simulink model "parte3_ex2"  (R2021b)
settings: Solver=VariableStepAuto  StartTime=0.0  StopTime=10  RelTol=1e-3
values from neighbouring files (symbols this model uses):
  h = 0.03    [parte3_script.m]
  Jm = 1.3475e-6    (= 1.3475e-06)    [parte3_script.m]
  Ke = 0.0159    [parte3_script.m]
  Kf = 0.000001176    (= 1.176e-06)    [parte3_script.m]
  L = Laa(2:end)    [parte3_script.m]
  L1 = -Laa(1)    [parte3_script.m]
  La = 0    [parte3_script.m]
  Lc = L1/(1-polo_i)    [parte3_script.m]
  Ra = 8    [parte3_script.m]
undefined symbols (not defined in the file or in its folder): DiscIntNeverNeededParam
settings Model: Creator=Dylan  LastModifiedBy=Dylan

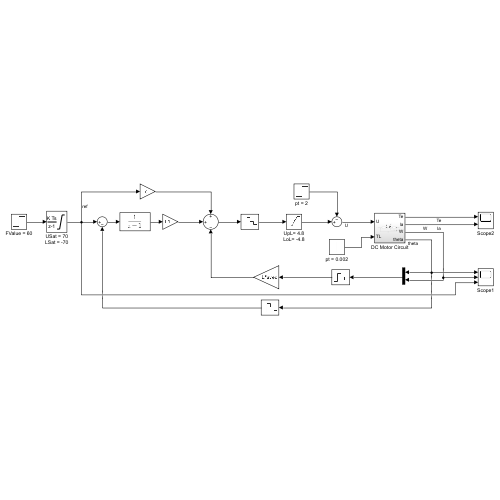
[thumbnail: Simulink's stored preview of the top-level diagram]
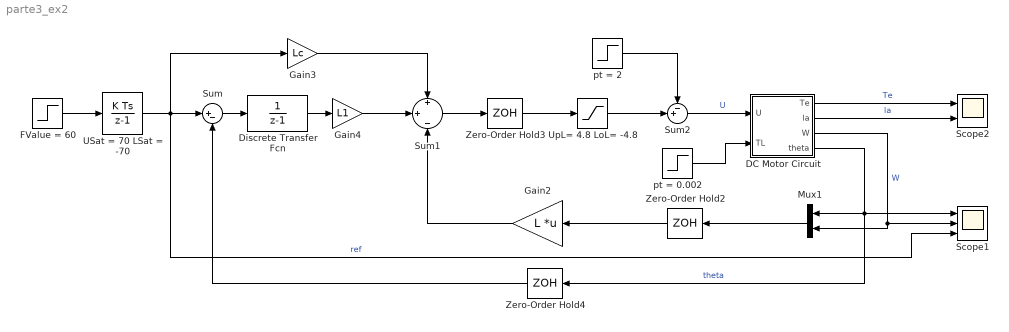
== system parte3_ex2 ==
  DC Motor Circuit : Subsystem
  Discrete Transfer Fcn : DiscreteTransferFcn  Denominator=[1 -1]  SampleTime=h
  FValue = 60 : Step  After=60  SampleTime=0
  Gain2 : Gain  Gain=L  Multiplication=Matrix(K*u) (u vector)
  Gain3 : Gain  Gain=Lc
  Gain4 : Gain  Gain=L1
  Mux1 : Mux  Inputs=2
  Scope1 : Scope  NumInputPorts=3
  Scope2 : Scope  NumInputPorts=2
  Sum : Sum  Inputs=|+-
  Sum1 : Sum  Inputs=+|+|-
  Sum2 : Sum  Inputs=-+|
  USat = 70 LSat = -70 : DiscreteIntegrator  SampleTime=h  LimitOutput=on  UpperSaturationLimit=70  LowerSaturationLimit=-70  ICPrevOutput=DiscIntNeverNeededParam  ICPrevScaledInput=DiscIntNeverNeededParam
  UpL= 4.8 LoL= -4.8 : Saturate  UpperLimit=4.8  LowerLimit=-4.8
  Zero-Order Hold2 : ZeroOrderHold  SampleTime=h
  Zero-Order Hold3 : ZeroOrderHold  SampleTime=h
  Zero-Order Hold4 : ZeroOrderHold  SampleTime=h
  pt = 0.002 : Step  Time=4  After=0.002  SampleTime=0
  pt = 2 : Step  Time=5  After=2  SampleTime=0
  wires:
  pt = 0.002/1 -> DC Motor Circuit/2(TL)
  FValue = 60/1 -> USat = 70 LSat = -70/1
  USat = 70 LSat = -70/1 -> Scope1/3, Sum/1, Gain3/1  "ref"
  Zero-Order Hold2/1 -> Gain2/1
  DC Motor Circuit/2(la) -> Scope2/2  "la"
  Sum1/1 -> Zero-Order Hold3/1
  Sum2/1 -> DC Motor Circuit/1(U)  "U"
  DC Motor Circuit/3(W) -> Mux1/2, Scope1/2  "W"
  Gain3/1 -> Sum1/1
  Mux1/1 -> Zero-Order Hold2/1
  DC Motor Circuit/1(Te) -> Scope2/1  "Te"
  Gain2/1 -> Sum1/3
  Gain4/1 -> Sum1/2
  Discrete Transfer Fcn/1 -> Gain4/1
  Sum/1 -> Discrete Transfer Fcn/1
  Zero-Order Hold4/1 -> Sum/2
  DC Motor Circuit/4(theta) -> Mux1/1, Scope1/1, Zero-Order Hold4/1  "theta"
  Zero-Order Hold3/1 -> UpL= 4.8 LoL= -4.8/1
  pt = 2/1 -> Sum2/1
  UpL= 4.8 LoL= -4.8/1 -> Sum2/2

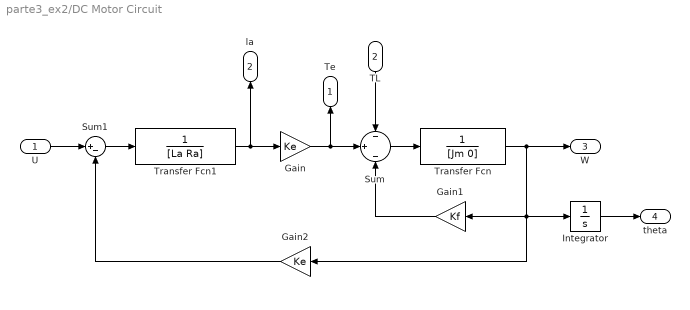
== system parte3_ex2/DC Motor Circuit ==
  U : Inport
  TL : Inport  Port=2
  Gain : Gain  Gain=Ke
  Gain1 : Gain  Gain=Kf
  Gain2 : Gain  Gain=Ke
  Integrator : Integrator
  Sum : Sum  Inputs=-|+|-
  Sum1 : Sum  Inputs=|+-
  Transfer Fcn : TransferFcn  Denominator=[Jm 0]
  Transfer Fcn1 : TransferFcn  Denominator=[La Ra]
  Te : Outport
  la : Outport  Port=2
  W : Outport  Port=3
  theta : Outport  Port=4
  wires:
  U/1 -> Sum1/1
  Transfer Fcn/1 -> W/1, Gain2/1, Integrator/1, Gain1/1
  Transfer Fcn1/1 -> la/1, Gain/1
  Gain2/1 -> Sum1/2
  Sum/1 -> Transfer Fcn/1
  Gain/1 -> Te/1, Sum/2
  TL/1 -> Sum/1
  Gain1/1 -> Sum/3
  Sum1/1 -> Transfer Fcn1/1
  Integrator/1 -> theta/1
